simulink model "flightControlSystem"  (R2021a)
settings: Solver=ode3  StartTime=0  StopTime=TFinal  FixedStep=Ts  RelTol=1e-3  EnableMultiTasking=on
undefined symbols (not defined in the file): landingAltitude, Ts
libraries: simulink x2
settings Model: Creator=The MathWorks, Inc.  LastModifiedBy=karol
settings SolverCC: AlgebraicLoopSolver=TrustRegion
settings DataIOCC: LimitDataPoints=on  SaveFormat=StructureWithTime  ReturnWorkspaceOutputs=off
settings OptimizationCC: BlockReduction=off  DefaultParameterBehavior=Inlined  BufferReuse=off  PassReuseOutputArgsThreshold=0
settings DebuggingCC: AlgebraicLoopMsg=none  IntegerOverflowMsg=none  ParameterPrecisionLossMsg=none  ParameterTunabilityLossMsg=error  UnconnectedInputMsg=none  UnconnectedOutputMsg=none  UnconnectedLineMsg=none  BusObjectLabelMismatch=error  SFUnexpectedBacktrackingDiag=warning  SFNoUnconditionalDefaultTransitionDiag=warning  SFExecutionAtInitializationDiag=none  SFMachineParentedDataDiag=warning  IntegerSaturationMsg=none  ArithmeticOperatorsInVariantConditions=warning
settings HardwareCC: ProdBitPerPointer=32  ProdBitPerSizeT=32  ProdBitPerPtrDiffT=32  ProdLargestAtomicInteger=Long  ProdWordSize=32  ProdHWDeviceType=ARM Compatible->ARM 9
settings ModelReferenceCC: ModelReferenceNumInstancesAllowed=Single  PropagateSignalLabelsOutOfModel=off
settings SFSimCC: SimUseLocalCustomCode=off  CustomCodeUndefinedFunction=UseInterfaceOnly
settings RTWCC: Description=Generic Real-Time Target  GenCodeOnly=on  PackageGeneratedCodeAndArtifacts=on  PackageName=FlightControllerFiles  GenerateReport=on  RTWUseLocalCustomCode=off  LaunchReport=on
settings CodeAppCC: ForceParamTrailComments=on  MaxIdLength=63  OperatorAnnotations=on  StateflowObjectComments=on  MATLABSourceComments=on
settings GRTTargetCC: TargetLangStandard=C89/C90 (ANSI)
settings ConfigComp: CovMetricSettings=dw  CovSaveCumulativeToWorkspaceVar=on  CovSaveSingleToWorkspaceVar=on  CovExternalEMLEnable=off  CovSFcnEnable=off

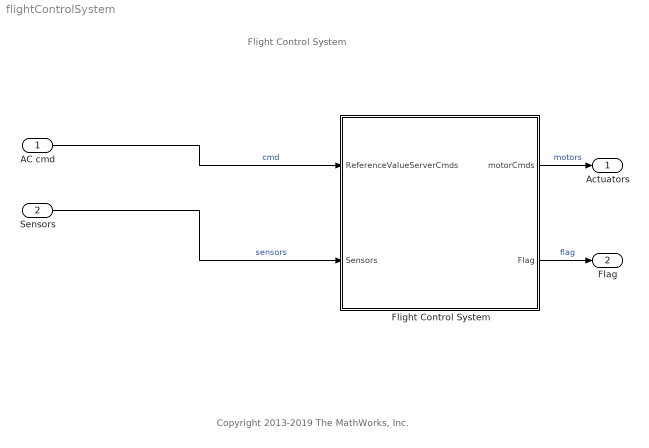
== system flightControlSystem ==
  note: Copyright 2013-2019 The MathWorks, Inc.
  note: Flight Control System
  AC cmd : Inport  OutDataTypeStr=Bus: CommandBus  BusOutputAsStruct=on
  Sensors : Inport  Port=2  OutDataTypeStr=Bus: SensorsBus  BusOutputAsStruct=on
  Flight Control System : Subsystem  TreatAsAtomicUnit=on  SystemSampleTime=Ts
  Actuators : Outport  OutDataTypeStr=single  PortDimensions=4  VectorParamsAs1DForOutWhenUnconnected=off
  Flag : Outport  Port=2  OutDataTypeStr=uint8  PortDimensions=1  VectorParamsAs1DForOutWhenUnconnected=off
  wires:
  AC cmd/1 -> Flight Control System/1(ReferenceValueServerCmds)  "cmd"
  Flight Control System/1(motorCmds) -> Actuators/1  "motors"
  Sensors/1 -> Flight Control System/2(Sensors)  "sensors"
  Flight Control System/2(Flag) -> Flag/1  "flag"

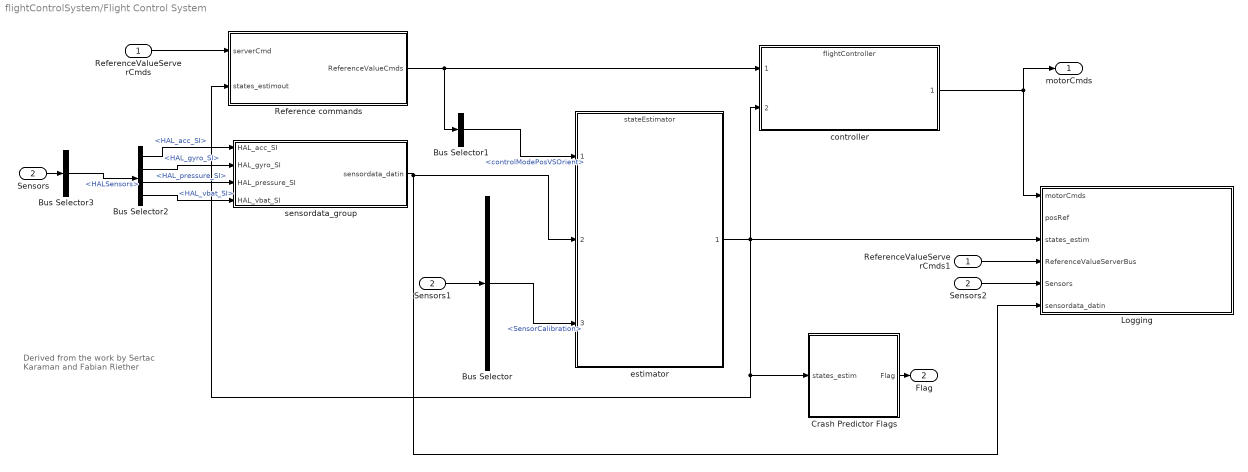
== system flightControlSystem/Flight Control System ==
  note: Derived from the work by Sertac
      | Karaman and Fabian Riether
  ReferenceValueServerCmds : Inport  OutDataTypeStr=Bus: CommandBus
  Sensors : Inport  Port=2  OutDataTypeStr=Bus: SensorsBus  BusOutputAsStruct=on
  Bus Selector : BusSelector  OutputSignals=SensorCalibration
  Bus Selector1 : BusSelector  OutputSignals=controlModePosVSOrient
  Bus Selector2 : BusSelector  OutputSignals=HAL_acc_SI,HAL_gyro_SI,HAL_pressure_SI,HAL_vbat_SI
  Bus Selector3 : BusSelector  OutputSignals=HALSensors
  Crash Predictor Flags : Subsystem
  Logging : Subsystem  TreatAsAtomicUnit=on
      settings: RTWFcnNameOpts=Use subsystem name
  Reference commands : Subsystem
  ReferenceValueServerCmds1 : InportShadow  OutDataTypeStr=Bus: CommandBus
  Sensors1 : InportShadow  Port=2  OutDataTypeStr=Bus: SensorsBus  BusOutputAsStruct=on
  Sensors2 : InportShadow  Port=2  OutDataTypeStr=Bus: SensorsBus  BusOutputAsStruct=on
  controller : ModelReference  ModelNameDialog=flightController.slx  SimulationMode=Normal  ModelReferenceVersion=4.2
  estimator : ModelReference  ModelNameDialog=stateEstimator.slx  SimulationMode=Normal  ModelReferenceVersion=4.8
  sensordata_group : Subsystem
  motorCmds : Outport  VectorParamsAs1DForOutWhenUnconnected=off
  Flag : Outport  Port=2  VectorParamsAs1DForOutWhenUnconnected=off
  wires:
  ReferenceValueServerCmds/1 -> Reference commands/1(serverCmd)
  Bus Selector2/1 -> sensordata_group/1(HAL_acc_SI)  "<HAL_acc_SI>"
  Bus Selector2/2 -> sensordata_group/2(HAL_gyro_SI)  "<HAL_gyro_SI>"
  estimator/1 -> Reference commands/2(states_estimout), Crash Predictor Flags/1(states_estim), Logging/3(states_estim), controller/2
  Sensors2/1 -> Logging/5(Sensors)
  ReferenceValueServerCmds1/1 -> Logging/4(ReferenceValueServerBus)
  controller/1 -> motorCmds/1, Logging/1(motorCmds)
  sensordata_group/1(sensordata_datin) -> Logging/6(sensordata_datin), estimator/2
  Bus Selector2/4 -> sensordata_group/4(HAL_vbat_SI)  "<HAL_vbat_SI>"
  Crash Predictor Flags/1(Flag) -> Flag/1
  Sensors/1 -> Bus Selector3/1
  Bus Selector3/1 -> Bus Selector2/1  "<HALSensors>"
  Sensors1/1 -> Bus Selector/1
  Bus Selector/1 -> estimator/3  "<SensorCalibration>"
  Bus Selector1/1 -> estimator/1  "<controlModePosVSOrient>"
  Reference commands/1(ReferenceValueCmds) -> Bus Selector1/1, controller/1
  Bus Selector2/3 -> sensordata_group/3(HAL_pressure_SI)  "<HAL_pressure_SI>"

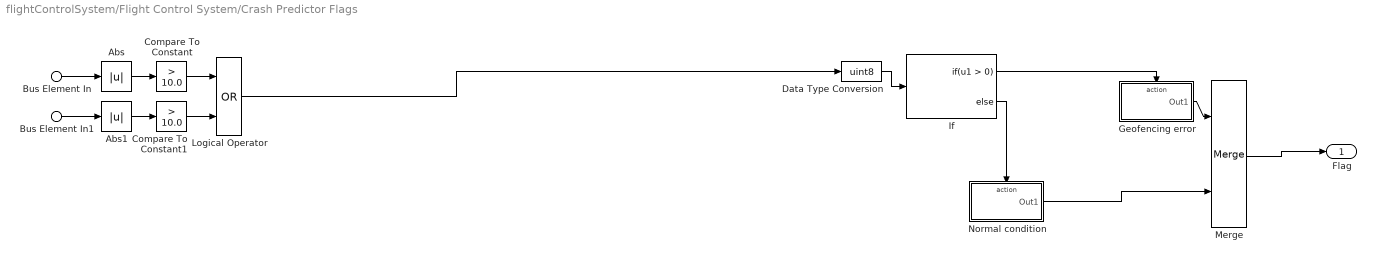
== system flightControlSystem/Flight Control System/Crash Predictor Flags ==
  Bus Element In : Inport  PortName=states_estim  Element=X
  Bus Element In1 : Inport  PortName=states_estim  Element=Y
  Abs : Abs
  Abs1 : Abs
  Compare To Constant : simulink/Logic and Bit Operations/Compare To Constant  relop=>  const=10.0  OutDataTypeStr=boolean
  Compare To Constant1 : simulink/Logic and Bit Operations/Compare To Constant  relop=>  const=10.0  OutDataTypeStr=boolean
  Data Type Conversion : DataTypeConversion  OutDataTypeStr=uint8  RndMeth=Nearest
  Geofencing error : Subsystem  TreatAsAtomicUnit=on
  If : If
  Logical Operator : Logic  Operator=OR  AllPortsSameDT=off
  Merge : Merge  InitialOutput=0
  Normal condition : Subsystem  TreatAsAtomicUnit=on
  Flag : Outport  VectorParamsAs1DForOutWhenUnconnected=off
  wires:
  Bus Element In/1 -> Abs/1
  Bus Element In1/1 -> Abs1/1
  Compare To Constant/1 -> Logical Operator/1
  Compare To Constant1/1 -> Logical Operator/2
  Abs/1 -> Compare To Constant/1
  Abs1/1 -> Compare To Constant1/1
  Logical Operator/1 -> Data Type Conversion/1
  Merge/1 -> Flag/1
  If/1 -> Geofencing error/Action
  If/2 -> Normal condition/Action
  Geofencing error/1(Out1) -> Merge/1
  Normal condition/1(Out1) -> Merge/2
  Data Type Conversion/1 -> If/1

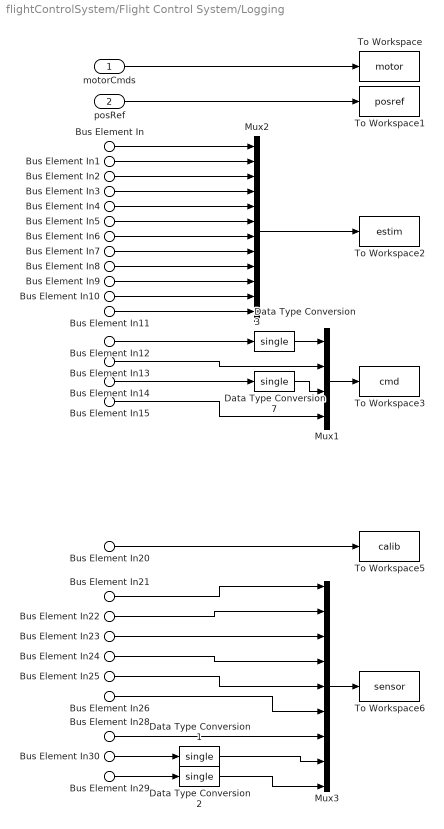
== system flightControlSystem/Flight Control System/Logging ==
  motorCmds : Inport
  posRef : Inport  Port=2
  Bus Element In : Inport  Port=3  PortName=states_estim  Element=X
  Bus Element In1 : Inport  Port=3  PortName=states_estim  Element=Y
  Bus Element In2 : Inport  Port=3  PortName=states_estim  Element=Z
  Bus Element In3 : Inport  Port=3  PortName=states_estim  Element=yaw
  Bus Element In6 : Inport  Port=3  PortName=states_estim  Element=dx
  Bus Element In5 : Inport  Port=3  PortName=states_estim  Element=roll
  Bus Element In4 : Inport  Port=3  PortName=states_estim  Element=pitch
  Bus Element In7 : Inport  Port=3  PortName=states_estim  Element=dy
  Bus Element In8 : Inport  Port=3  PortName=states_estim  Element=dz
  Bus Element In9 : Inport  Port=3  PortName=states_estim  Element=p
  Bus Element In10 : Inport  Port=3  PortName=states_estim  Element=q
  Bus Element In11 : Inport  Port=3  PortName=states_estim  Element=r
  Bus Element In12 : Inport  Port=4  PortName=ReferenceValueServerBus  Element=controlModePosVSOrient
  Bus Element In13 : Inport  Port=4  PortName=ReferenceValueServerBus  Element=pos_ref
  Bus Element In14 : Inport  Port=4  PortName=ReferenceValueServerBus  Element=takeoff_flag
  Bus Element In15 : Inport  Port=4  PortName=ReferenceValueServerBus  Element=orient_ref
  Bus Element In20 : Inport  Port=5  PortName=Sensors  Element=SensorCalibration
  Bus Element In21 : Inport  Port=6  PortName=sensordata_datin  Element=ddx
  Bus Element In22 : Inport  Port=6  PortName=sensordata_datin  Element=ddy
  Bus Element In23 : Inport  Port=6  PortName=sensordata_datin  Element=ddz
  Bus Element In24 : Inport  Port=6  PortName=sensordata_datin  Element=p
  Bus Element In25 : Inport  Port=6  PortName=sensordata_datin  Element=q
  Bus Element In26 : Inport  Port=6  PortName=sensordata_datin  Element=r
  Bus Element In28 : Inport  Port=6  PortName=sensordata_datin  Element=prs
  Bus Element In29 : Inport  Port=6  PortName=sensordata_datin  Element=vbat_percentage
  Bus Element In30 : Inport  Port=6  PortName=sensordata_datin  Element=vbat_V
  Data Type Conversion{1..3,7} (4 alike) : DataTypeConversion  OutDataTypeStr=single
  Mux1 : Mux
  Mux2 : Mux  Inputs=12
  Mux3 : Mux  Inputs=9
  To Workspace : ToWorkspace  VariableName=motor  SaveFormat=Structure With Time  SampleTime=-1
  To Workspace1 : ToWorkspace  VariableName=posref  SaveFormat=Structure With Time  SampleTime=-1
  To Workspace2 : ToWorkspace  VariableName=estim  SaveFormat=Structure With Time  SampleTime=-1
  To Workspace3 : ToWorkspace  VariableName=cmd  SaveFormat=Structure With Time  SampleTime=-1
  To Workspace5 : ToWorkspace  VariableName=calib  SaveFormat=Structure With Time  SampleTime=-1
      settings: Decimation=100
  To Workspace6 : ToWorkspace  VariableName=sensor  SaveFormat=Structure With Time  SampleTime=-1
  wires:
  Bus Element In12/1 -> Data Type Conversion3/1
  Bus Element In14/1 -> Data Type Conversion7/1
  Bus Element In20/1 -> To Workspace5/1
  Mux2/1 -> To Workspace2/1
  motorCmds/1 -> To Workspace/1
  Mux1/1 -> To Workspace3/1
  Bus Element In3/1 -> Mux2/4
  Bus Element In5/1 -> Mux2/6
  Bus Element In4/1 -> Mux2/5
  Bus Element In8/1 -> Mux2/9
  Bus Element In6/1 -> Mux2/7
  Bus Element In7/1 -> Mux2/8
  Bus Element In9/1 -> Mux2/10
  Bus Element In11/1 -> Mux2/12
  Bus Element In1/1 -> Mux2/2
  Bus Element In10/1 -> Mux2/11
  Bus Element In2/1 -> Mux2/3
  Bus Element In/1 -> Mux2/1
  Data Type Conversion3/1 -> Mux1/1
  Bus Element In13/1 -> Mux1/2
  Data Type Conversion7/1 -> Mux1/3
  Bus Element In15/1 -> Mux1/4
  posRef/1 -> To Workspace1/1
  Bus Element In21/1 -> Mux3/1
  Bus Element In22/1 -> Mux3/2
  Bus Element In23/1 -> Mux3/3
  Bus Element In24/1 -> Mux3/4
  Bus Element In25/1 -> Mux3/5
  Bus Element In26/1 -> Mux3/6
  Bus Element In30/1 -> Data Type Conversion1/1
  Bus Element In29/1 -> Data Type Conversion2/1
  Mux3/1 -> To Workspace6/1
  Data Type Conversion1/1 -> Mux3/8
  Data Type Conversion2/1 -> Mux3/9
  Bus Element In28/1 -> Mux3/7

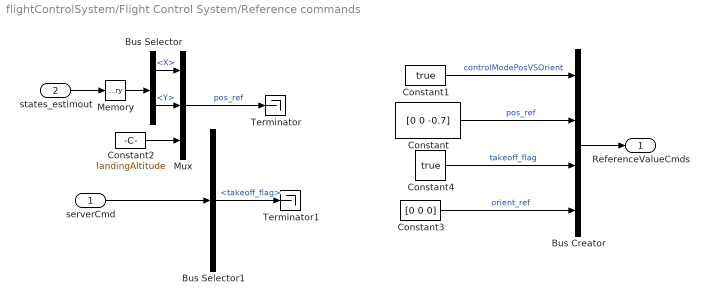
== system flightControlSystem/Flight Control System/Reference commands ==
  serverCmd : Inport
  states_estimout : Inport  Port=2
  Bus Creator : BusCreator  Inputs=4  OutDataTypeStr=Bus: CommandBus  NonVirtualBus=on
  Bus Selector : BusSelector  OutputSignals=X,Y
  Bus Selector1 : BusSelector  OutputSignals=takeoff_flag
  Constant : Constant  Value=[0 0 -0.7]  OutDataTypeStr=single
  Constant1 : Constant  Value=true  OutDataTypeStr=boolean
  Constant2 : Constant  Value=landingAltitude  OutDataTypeStr=single
  Constant3 : Constant  Value=[0 0 0]  OutDataTypeStr=single
  Constant4 : Constant  Value=true  OutDataTypeStr=boolean
  Memory : Memory  InheritSampleTime=on
  Mux : Mux  Inputs=3
  Terminator : Terminator
  Terminator1 : Terminator
  ReferenceValueCmds : Outport  OutDataTypeStr=Bus: CommandBus  VectorParamsAs1DForOutWhenUnconnected=off
  wires:
  Mux/1 -> Terminator/1  "pos_ref"
  Constant1/1 -> Bus Creator/1  "controlModePosVSOrient"
  Bus Selector1/1 -> Terminator1/1  "<takeoff_flag>"
  states_estimout/1 -> Memory/1
  Bus Selector/1 -> Mux/1  "<X>"
  Constant2/1 -> Mux/3
  Bus Selector/2 -> Mux/2  "<Y>"
  serverCmd/1 -> Bus Selector1/1
  Constant3/1 -> Bus Creator/4  "orient_ref"
  Memory/1 -> Bus Selector/1
  Bus Creator/1 -> ReferenceValueCmds/1
  Constant/1 -> Bus Creator/2  "pos_ref"
  Constant4/1 -> Bus Creator/3  "takeoff_flag"

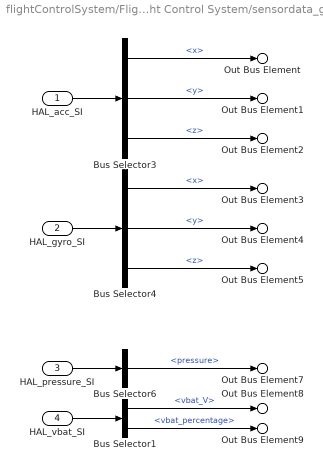
== system flightControlSystem/Flight Control System/sensordata_group ==
  HAL_acc_SI : Inport  OutDataTypeStr=Bus: HAL_acc_SI_t
  HAL_gyro_SI : Inport  Port=2  OutDataTypeStr=Bus: HAL_gyro_SI_t
  HAL_pressure_SI : Inport  Port=3  OutDataTypeStr=Bus: HAL_pressure_SI_t
  HAL_vbat_SI : Inport  Port=4  OutDataTypeStr=Bus: HAL_vbat_SI_t
  Bus Selector1 : BusSelector  OutputSignals=vbat_V,vbat_percentage
  Bus Selector3 : BusSelector  OutputSignals=x,y,z
  Bus Selector4 : BusSelector  OutputSignals=x,y,z
  Bus Selector6 : BusSelector  OutputSignals=pressure
  Out Bus Element : Outport  VectorParamsAs1DForOutWhenUnconnected=off  PortName=sensordata_datin  Element=ddx
  Out Bus Element1 : Outport  VectorParamsAs1DForOutWhenUnconnected=off  PortName=sensordata_datin  Element=ddy
  Out Bus Element2 : Outport  VectorParamsAs1DForOutWhenUnconnected=off  PortName=sensordata_datin  Element=ddz
  Out Bus Element3 : Outport  VectorParamsAs1DForOutWhenUnconnected=off  PortName=sensordata_datin  Element=p
  Out Bus Element4 : Outport  VectorParamsAs1DForOutWhenUnconnected=off  PortName=sensordata_datin  Element=q
  Out Bus Element5 : Outport  VectorParamsAs1DForOutWhenUnconnected=off  PortName=sensordata_datin  Element=r
  Out Bus Element7 : Outport  VectorParamsAs1DForOutWhenUnconnected=off  PortName=sensordata_datin  Element=prs
  Out Bus Element8 : Outport  VectorParamsAs1DForOutWhenUnconnected=off  PortName=sensordata_datin  Element=vbat_V
  Out Bus Element9 : Outport  VectorParamsAs1DForOutWhenUnconnected=off  PortName=sensordata_datin  Element=vbat_percentage
  wires:
  HAL_gyro_SI/1 -> Bus Selector4/1
  HAL_acc_SI/1 -> Bus Selector3/1
  HAL_pressure_SI/1 -> Bus Selector6/1
  Bus Selector4/1 -> Out Bus Element3/1  "<x>"
  Bus Selector3/3 -> Out Bus Element2/1  "<z>"
  Bus Selector4/3 -> Out Bus Element5/1  "<z>"
  Bus Selector6/1 -> Out Bus Element7/1  "<pressure>"
  Bus Selector4/2 -> Out Bus Element4/1  "<y>"
  Bus Selector3/1 -> Out Bus Element/1  "<x>"
  Bus Selector3/2 -> Out Bus Element1/1  "<y>"
  Bus Selector1/1 -> Out Bus Element8/1  "<vbat_V>"
  HAL_vbat_SI/1 -> Bus Selector1/1
  Bus Selector1/2 -> Out Bus Element9/1  "<vbat_percentage>"

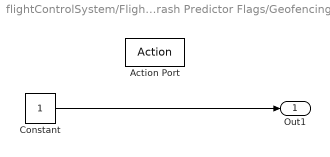
== system flightControlSystem/Flight Control System/Crash Predictor Flags/Geofencing error ==
  Action Port : ActionPort  ActionPortLabel=if(u1 > 0)
  Constant : Constant  OutDataTypeStr=uint8
  Out1 : Outport  VectorParamsAs1DForOutWhenUnconnected=off
  wires:
  Constant/1 -> Out1/1

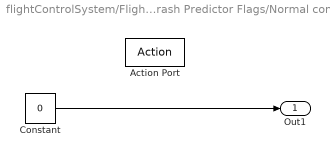
== system flightControlSystem/Flight Control System/Crash Predictor Flags/Normal condition ==
  Action Port : ActionPort  ActionPortLabel=else
  Constant : Constant  Value=0  OutDataTypeStr=uint8
  Out1 : Outport  VectorParamsAs1DForOutWhenUnconnected=off
  wires:
  Constant/1 -> Out1/1
